simulink model "sl_subsys_fcncall2"  (Simulink 6.0)
settings: Solver=FixedStepDiscrete  StartTime=0.0  StopTime=10.0  FixedStep=1  RelTol=1e-3
settings Model: CovMetricSettings=d  Creator=The MathWorks Inc.  LastModifiedBy=batserve  ExtModeAutoUpdateStatusClock=off
settings OptimizationCC: BlockReduction=off  BooleanDataType=off
settings DebuggingCC: CheckExecutionContextPreStartOutputMsg=on  CheckExecutionContextRuntimeOutputMsg=on  SolverPrmCheckMsg=none
settings HardwareCC: TargetUnknown=on

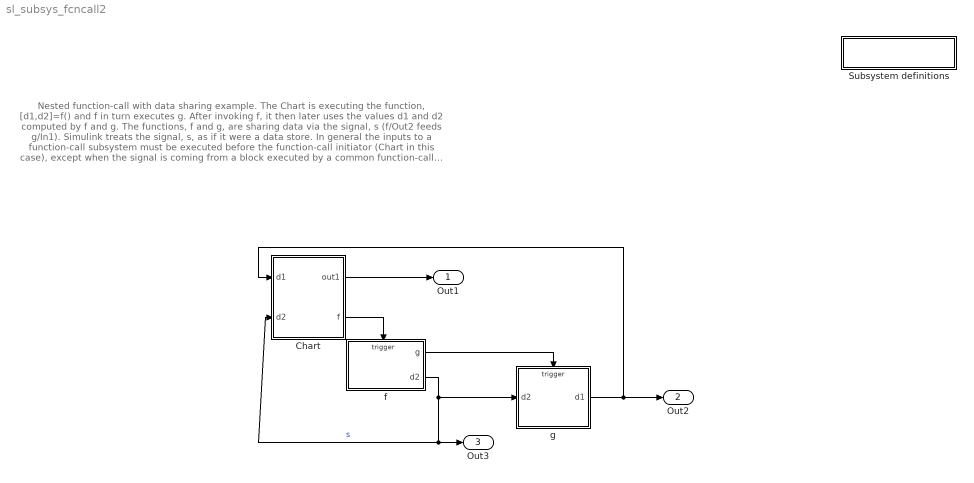
== system sl_subsys_fcncall2 ==
  note: Nested function-call with data sharing example.
      |
      | The Chart is executing the function, [d1,d2]=f() and f in turn executes g.
      | After invoking f, it then later uses the values d1 and d2 computed by f and g.
      | The functions, f and g, are sharing data via the signal, s (f/Out2 feeds g/In1).
      | Simulink treats the signal, s, as if it were a data store.
      |
      | In general the inputs to a function-call subsystem must be executed before the
      | function-call initiator (Chart in this case), except when the signal is coming
      | from a block executed by a common function-call initiator. For our example,
      | f() is a function-call initiator of g(). However Chart is a function-call
      | initiator of f(), thus Chart is a common function-call initiator of both
      | f() and g(). Therefore, the signal, s, below can be thought of as a data store in
      | that it is like a global working variable that is read and written to by
      | f() and g() in any given order (as defined by the Chart).
  " Subsystem definitions" : Subsystem  PropExecContextAcrossSSBoundary=on
      settings: OpenFcn=helpview([matlabroot,'/toolbox/simulink/simdemos/sl_subsys_definitions.html']);
      mask Display: disp('Subsystem\ndefinitions')
  Chart : Stateflow chart  PropExecContextAcrossSSBoundary=on
  f : Subsystem  TreatAsAtomicUnit=on  PropExecContextAcrossSSBoundary=on
  g : Subsystem  TreatAsAtomicUnit=on  PropExecContextAcrossSSBoundary=on
  Out1 : Outport
  Out2 : Outport  Port=2
  Out3 : Outport  Port=3
  wires:
  Chart/2(f) -> f/Trigger
  f/1(g) -> g/Trigger
  f/2(d2) -> Out3/1, Chart/2(d2), g/1(d2)  "s"
  g/1(d1) -> Out2/1, Chart/1(d1)
  Chart/1(out1) -> Out1/1

== system sl_subsys_fcncall2/ Subsystem definitions ==

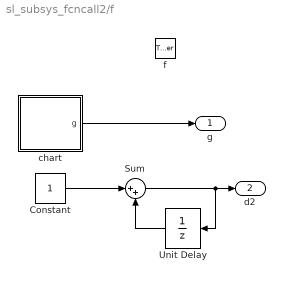
== system sl_subsys_fcncall2/f ==
  f : TriggerPort  TriggerType=function-call
  Constant : Constant
  Sum : Sum  Inputs=|++  SaturateOnIntegerOverflow=on  InputSameDT=on
  Unit Delay : UnitDelay  Orientation=left  SampleTime=-1
  chart : Stateflow chart  PropExecContextAcrossSSBoundary=on
  g : Outport
  d2 : Outport  Port=2
  wires:
  chart/1(g) -> g/1
  Constant/1 -> Sum/1
  Unit Delay/1 -> Sum/2
  Sum/1 -> d2/1, Unit Delay/1

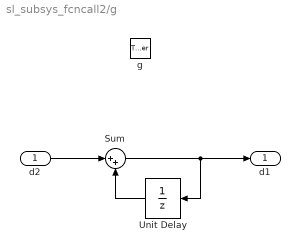
== system sl_subsys_fcncall2/g ==
  d2 : Inport  Port=1  LatchInput=off
  g : TriggerPort  TriggerType=function-call
  Sum : Sum  Inputs=|++  SaturateOnIntegerOverflow=on  InputSameDT=on
  Unit Delay : UnitDelay  Orientation=left  SampleTime=-1
  d1 : Outport
  wires:
  d2/1 -> Sum/1
  Unit Delay/1 -> Sum/2
  Sum/1 -> d1/1, Unit Delay/1

== stateflow chart Chart ==
  state one/
    entry:f;out1=d1+d2;
  state two/
    entry: f;out1=d1-d2;
  one -> two
  two -> one
  (default) -> one
  data: d1 input double; d2 input double; out1 output double; out local double
  events: f output FUNCTION_CALL_EVENT

== stateflow chart f/chart ==
  state one/
    entry: g;
  state two/
    entry: g;
  one -> two
  two -> one
  (default) -> one
  events: g output FUNCTION_CALL_EVENT
